simulink model "Simulink_mg_1234_with_DistributedControl_ControlConmutado"  (R2018a)
settings: Solver=VariableStepAuto  StartTime=0.0  StopTime=50  FixedStep=1e-6  MaxStep=1e-3  RelTol=1e-3
values from neighbouring files (symbols this model uses):
  aij = 1    [Simulation_Base_4_mg.m]    (also in Simulation_alpha_vs_tau.m)
  aij_1 = 10    [Simulation_Base_4_mg.m]    (also in Simulation_alpha_vs_tau.m)
  aij_2 = 10    [Simulation_Base_4_mg.m]    (also in Simulation_alpha_vs_tau.m)
  aij_3 = 10    [Simulation_Base_4_mg.m]    (also in Simulation_alpha_vs_tau.m)
  aij_4 = 10    [Simulation_Base_4_mg.m]    (also in Simulation_alpha_vs_tau.m)
  C_mg_1 = Ctot .* dist    [Simulation_Base_4_mg.m]    (also in Simulation_alpha_vs_tau.m)
  C_mg_2 = Ctot .* dist    [Simulation_Base_4_mg.m]    (also in Simulation_alpha_vs_tau.m)
  C_mg_3 = Ctot .* dist    [Simulation_Base_4_mg.m]    (also in Simulation_alpha_vs_tau.m)
  C_mg_4 = Ctot .* dist    [Simulation_Base_4_mg.m]    (also in Simulation_alpha_vs_tau.m)
  g12 = 1.2    [Simulation_Base_4_mg.m]    (also in Simulation_alpha_vs_tau.m)
  g12_1 = 1/r_jk    (= 10)    [Simulation_Base_4_mg.m]    (also in Simulation_alpha_vs_tau.m)
  g12_2 = 1/r_jk    (= 10)    [Simulation_Base_4_mg.m]    (also in Simulation_alpha_vs_tau.m)
  g12_3 = 1/r_jk    (= 10)    [Simulation_Base_4_mg.m]    (also in Simulation_alpha_vs_tau.m)
  g12_4 = 1/r_jk    (= 10)    [Simulation_Base_4_mg.m]    (also in Simulation_alpha_vs_tau.m)
  g13 = ((0.383+1.756) / (0.383*1.756))^(-1)    (= 0.31442169238)    [Simulation_Base_4_mg.m]    (also in Simulation_alpha_vs_tau.m)
  g13_1 = 1/r_jk    (= 10)    [Simulation_Base_4_mg.m]    (also in Simulation_alpha_vs_tau.m)
  g13_3 = 1/r_jk    (= 10)    [Simulation_Base_4_mg.m]    (also in Simulation_alpha_vs_tau.m)
  g13_4 = 1/r_jk    (= 10)    [Simulation_Base_4_mg.m]    (also in Simulation_alpha_vs_tau.m)
  g23_1 = 1/r_jk    (= 10)    [Simulation_Base_4_mg.m]    (also in Simulation_alpha_vs_tau.m)
  g23_4 = 1/r_jk    (= 10)    [Simulation_Base_4_mg.m]    (also in Simulation_alpha_vs_tau.m)
  g24 = 1.55    [Simulation_Base_4_mg.m]    (also in Simulation_alpha_vs_tau.m)
  g24_3 = 1/r_jk    (= 10)    [Simulation_Base_4_mg.m]    (also in Simulation_alpha_vs_tau.m)
  g24_4 = 1/r_jk    (= 10)    [Simulation_Base_4_mg.m]    (also in Simulation_alpha_vs_tau.m)
  g34 = 0.75    [Simulation_Base_4_mg.m]    (also in Simulation_alpha_vs_tau.m)
  g34_3 = 1/r_jk    (= 10)    [Simulation_Base_4_mg.m]    (also in Simulation_alpha_vs_tau.m)
  g34_4 = 1/r_jk    (= 10)    [Simulation_Base_4_mg.m]    (also in Simulation_alpha_vs_tau.m)
  h = 0.99    [Simulation_Base_4_mg.m]    (also in Simulation_alpha_vs_tau.m)
  I_rate = [100,50,33,33]    [Simulation_Base_4_mg.m]    (also in Simulation_alpha_vs_tau.m)
  I_rate_1 = [5, 2.5, 2.5]    [Simulation_Base_4_mg.m]    (also in Simulation_alpha_vs_tau.m)
  I_rate_2 = [2.5, 5]    [Simulation_Base_4_mg.m]    (also in Simulation_alpha_vs_tau.m)
  I_rate_3 = [4, 3, 2, 1]    [Simulation_Base_4_mg.m]    (also in Simulation_alpha_vs_tau.m)
  I_rate_4 = [4, 3, 2, 1]    [Simulation_Base_4_mg.m]    (also in Simulation_alpha_vs_tau.m)
  k_ii = 60    [Simulation_Base_4_mg.m]    (also in Simulation_alpha_vs_tau.m)
  k_ii2 = 10    [Simulation_Base_4_mg.m]    (also in Simulation_alpha_vs_tau.m)
  k_ii_1 = 1000    [Simulation_Base_4_mg.m]    (also in Simulation_alpha_vs_tau.m)
  k_ii_2 = 1000    [Simulation_Base_4_mg.m]    (also in Simulation_alpha_vs_tau.m)
  k_ii_3 = 1000    [Simulation_Base_4_mg.m]    (also in Simulation_alpha_vs_tau.m)
  k_ii_4 = 1000    [Simulation_Base_4_mg.m]    (also in Simulation_alpha_vs_tau.m)
  k_iv = 3    [Simulation_Base_4_mg.m]    (also in Simulation_alpha_vs_tau.m = 1)
  k_iv_1 = 30    [Simulation_Base_4_mg.m]    (also in Simulation_alpha_vs_tau.m)
  k_iv_2 = 30    [Simulation_Base_4_mg.m]    (also in Simulation_alpha_vs_tau.m)
  k_iv_3 = 30    [Simulation_Base_4_mg.m]    (also in Simulation_alpha_vs_tau.m)
  k_iv_4 = 30    [Simulation_Base_4_mg.m]    (also in Simulation_alpha_vs_tau.m)
  k_pi = 30    [Simulation_Base_4_mg.m]    (also in Simulation_alpha_vs_tau.m = 25)
  k_pi2 = 0.5    [Simulation_Base_4_mg.m]    (also in Simulation_alpha_vs_tau.m)
  k_pi_1 = 10    [Simulation_Base_4_mg.m]    (also in Simulation_alpha_vs_tau.m)
  k_pi_2 = 10    [Simulation_Base_4_mg.m]    (also in Simulation_alpha_vs_tau.m)
  k_pi_3 = 10    [Simulation_Base_4_mg.m]    (also in Simulation_alpha_vs_tau.m)
  k_pi_4 = 10    [Simulation_Base_4_mg.m]    (also in Simulation_alpha_vs_tau.m)
  kd_1 = [5, 2.5, 2.5]    [Simulation_Base_4_mg.m]    (also in Simulation_alpha_vs_tau.m)
  kd_2 = [2.5, 50]    [Simulation_Base_4_mg.m]    (also in Simulation_alpha_vs_tau.m)
  kd_3 = [4, 3, 2, 1]    [Simulation_Base_4_mg.m]    (also in Simulation_alpha_vs_tau.m)
  kd_4 = [4, 3, 2, 1]    [Simulation_Base_4_mg.m]    (also in Simulation_alpha_vs_tau.m)
  L_mg_1 = ones(n) .* n .* Ltot    [Simulation_Base_4_mg.m]    (also in Simulation_alpha_vs_tau.m)
  L_mg_2 = ones(n) .* n .* Ltot    [Simulation_Base_4_mg.m]    (also in Simulation_alpha_vs_tau.m)
  L_mg_3 = ones(n) .* n .* Ltot    [Simulation_Base_4_mg.m]    (also in Simulation_alpha_vs_tau.m)
  L_mg_4 = ones(n) .* n .* Ltot    [Simulation_Base_4_mg.m]    (also in Simulation_alpha_vs_tau.m)
  P_load_vertex_1 = [   P_load_vertex_1;                                                 P_aux(i1,1) , P_aux(i2,2) , P_aux(i3,3) ]    [Simulation_Base_4_mg.m]    (also in Simulation_alpha_vs_tau.m)
  P_load_vertex_2 = [   P_load_vertex_2;                                                 P_aux(i1,1) , P_aux(i2,2) ]    [Simulation_Base_4_mg.m]    (also in Simulation_alpha_vs_tau.m)
  P_load_vertex_3 = [   P_load_vertex_3;                                                 P_aux(i1,1) , P_aux(i2,2) , P_aux(i3,3), P_aux(i4,4) ]    [Simulation_Base_4_mg.m]    (also in Simulation_alpha_vs_tau.m)
  P_load_vertex_4 = [   P_load_vertex_4;                                                 P_aux(i1,1) , P_aux(i2,2) , P_aux(i3,3), P_aux(i4,4) ]    [Simulation_Base_4_mg.m]    (also in Simulation_alpha_vs_tau.m)
  r_d0 = 1.3    [Simulation_Base_4_mg.m]    (also in Simulation_alpha_vs_tau.m)
  rd_mg_1 = n^2 * rtot .* dist    [Simulation_Base_4_mg.m]    (also in Simulation_alpha_vs_tau.m)
  rd_mg_2 = n^2 * rtot .* dist    [Simulation_Base_4_mg.m]    (also in Simulation_alpha_vs_tau.m)
  rd_mg_3 = n^2 * rtot .* dist    [Simulation_Base_4_mg.m]    (also in Simulation_alpha_vs_tau.m)
  rd_mg_4 = n^2 * rtot .* dist    [Simulation_Base_4_mg.m]    (also in Simulation_alpha_vs_tau.m)
  tau = 0.5    [Simulation_Base_4_mg.m]    (also in Simulation_alpha_vs_tau.m = 0.066)
  time_1 = 0.5    [Simulation_Base_4_mg.m]    (also in Simulation_alpha_vs_tau.m)
  time_2 = 15    [Simulation_Base_4_mg.m]    (also in Simulation_alpha_vs_tau.m = 5)
  time_4 = 5    [Simulation_Base_4_mg.m]    (also in Simulation_alpha_vs_tau.m = 15)
  time_6 = 50    [Simulation_Base_4_mg.m]    (also in Simulation_alpha_vs_tau.m = 13)
  time_7 = 50    [Simulation_Base_4_mg.m]    (also in Simulation_alpha_vs_tau.m = 100)
  time_8 = 50    [Simulation_Base_4_mg.m]    (also in Simulation_alpha_vs_tau.m = 100)
  time_9 = 100    [Simulation_Base_4_mg.m]    (also in Simulation_alpha_vs_tau.m)
  time_a_down = 100    [Simulation_alpha_vs_tau.m]
  time_a_up = 100    [Simulation_alpha_vs_tau.m]
  time_tau_down = 25    [Simulation_alpha_vs_tau.m]
  V_ref = 1050    [Simulation_Base_4_mg.m]    (also in Simulation_alpha_vs_tau.m)
undefined symbols (not defined in the file or in its folder): Zout_den_source, Zout_num_source
libraries: fl_lib x128, nesl_utility x89, elec_lib x26
(part 2 of 2)

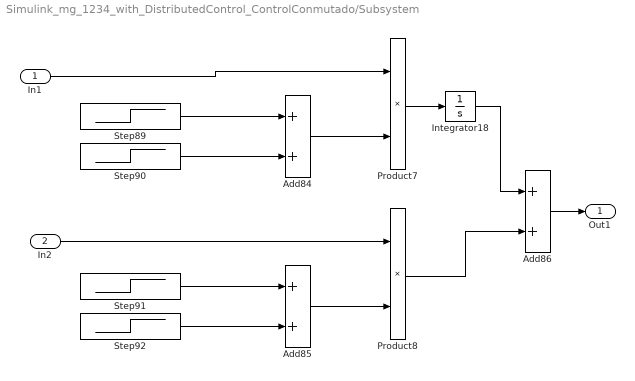
== system Simulink_mg_1234_with_DistributedControl_ControlConmutado/Subsystem ==
  In1 : Inport
  In2 : Inport  Port=2
  Add84 : Sum
  Add85 : Sum
  Add86 : Sum
  Integrator18 : Integrator
  Product7 : Product
  Product8 : Product
  Step89 : Step  Time=time_8  Before=k_ii  After=k_ii2  SampleTime=0
  Step90 : Step  Time=time_9  SampleTime=0
  Step91 : Step  Time=time_8  Before=k_pi  After=k_pi2  SampleTime=0
  Step92 : Step  Time=time_9  SampleTime=0
  Out1 : Outport
  wires:
  Integrator18/1 -> Add86/1
  Step92/1 -> Add85/2
  Add85/1 -> Product8/2
  Step89/1 -> Add84/1
  Step90/1 -> Add84/2
  Step91/1 -> Add85/1
  Add84/1 -> Product7/2
  Product7/1 -> Integrator18/1
  Product8/1 -> Add86/2
  In2/1 -> Product8/1
  In1/1 -> Product7/1
  Add86/1 -> Out1/1

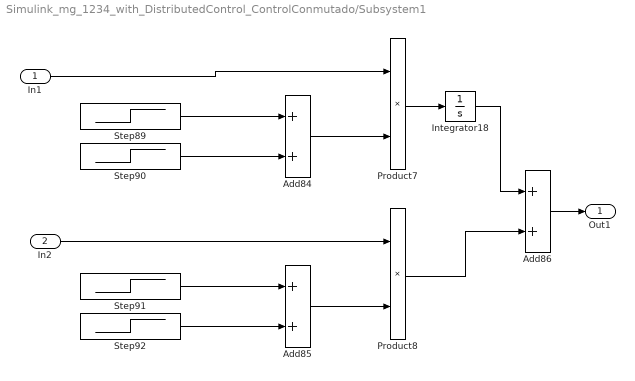
== system Simulink_mg_1234_with_DistributedControl_ControlConmutado/Subsystem1 ==
  In1 : Inport
  In2 : Inport  Port=2
  Add84 : Sum
  Add85 : Sum
  Add86 : Sum
  Integrator18 : Integrator
  Product7 : Product
  Product8 : Product
  Step89 : Step  Time=time_8  Before=k_ii  After=k_ii2  SampleTime=0
  Step90 : Step  Time=time_9  SampleTime=0
  Step91 : Step  Time=time_8  Before=k_pi  After=k_pi2  SampleTime=0
  Step92 : Step  Time=time_9  SampleTime=0
  Out1 : Outport
  wires:
  Add86/1 -> Out1/1
  In1/1 -> Product7/1
  In2/1 -> Product8/1
  Product8/1 -> Add86/2
  Product7/1 -> Integrator18/1
  Add84/1 -> Product7/2
  Step91/1 -> Add85/1
  Step90/1 -> Add84/2
  Step89/1 -> Add84/1
  Add85/1 -> Product8/2
  Step92/1 -> Add85/2
  Integrator18/1 -> Add86/1

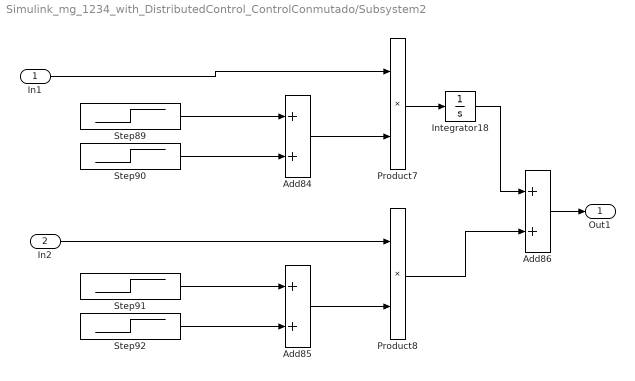
== system Simulink_mg_1234_with_DistributedControl_ControlConmutado/Subsystem2 ==
  In1 : Inport
  In2 : Inport  Port=2
  Add84 : Sum
  Add85 : Sum
  Add86 : Sum
  Integrator18 : Integrator
  Product7 : Product
  Product8 : Product
  Step89 : Step  Time=time_8  Before=k_ii  After=k_ii2  SampleTime=0
  Step90 : Step  Time=time_9  SampleTime=0
  Step91 : Step  Time=time_8  Before=k_pi  After=k_pi2  SampleTime=0
  Step92 : Step  Time=time_9  SampleTime=0
  Out1 : Outport
  wires:
  Add86/1 -> Out1/1
  In1/1 -> Product7/1
  In2/1 -> Product8/1
  Product8/1 -> Add86/2
  Product7/1 -> Integrator18/1
  Add84/1 -> Product7/2
  Step91/1 -> Add85/1
  Step90/1 -> Add84/2
  Step89/1 -> Add84/1
  Add85/1 -> Product8/2
  Step92/1 -> Add85/2
  Integrator18/1 -> Add86/1

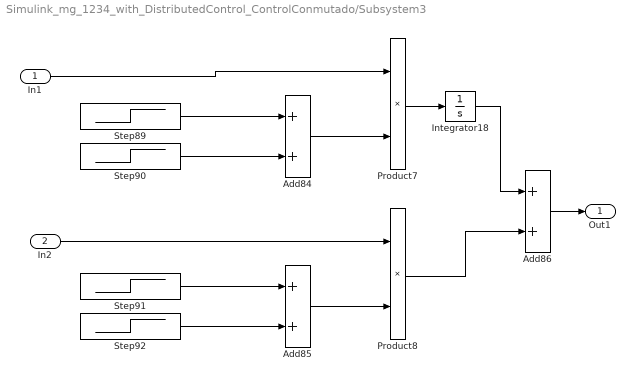
== system Simulink_mg_1234_with_DistributedControl_ControlConmutado/Subsystem3 ==
  In1 : Inport
  In2 : Inport  Port=2
  Add84 : Sum
  Add85 : Sum
  Add86 : Sum
  Integrator18 : Integrator
  Product7 : Product
  Product8 : Product
  Step89 : Step  Time=time_8  Before=k_ii  After=k_ii2  SampleTime=0
  Step90 : Step  Time=time_9  SampleTime=0
  Step91 : Step  Time=time_8  Before=k_pi  After=k_pi2  SampleTime=0
  Step92 : Step  Time=time_9  SampleTime=0
  Out1 : Outport
  wires:
  Integrator18/1 -> Add86/1
  Step92/1 -> Add85/2
  Add85/1 -> Product8/2
  Step89/1 -> Add84/1
  Step90/1 -> Add84/2
  Step91/1 -> Add85/1
  Add84/1 -> Product7/2
  Product7/1 -> Integrator18/1
  Product8/1 -> Add86/2
  In2/1 -> Product8/1
  In1/1 -> Product7/1
  Add86/1 -> Out1/1

== matlab function Simulink_mg_1234_with_DistributedControl_ControlConmutado/MATLAB Function1 ==
  data: i input; error_1 output; error_2 output; error_3 output; error_4 output; aij input
function [error_1,error_2,error_3, error_4] = fcn(i, aij)


%aij = 30;
%Connection matrix
AG = [  0 aij aij aij ; ...
        aij 0 aij aij ; ...
        aij aij 0 aij ;...
        aij aij aij 0]; %Communication matrices
n = 4;
i_int = i';
AG1 = AG - eye(n);
%sum_a = sum(AG1');
sum_a = sum(AG');
%AG1 = AG1 * i_int';
AG = AG * i_int';


%error = sum_a .* i_int - AG1';
error = sum_a .* i_int - AG';
error_1 = -error(1); 
error_2 = -error(2);
error_3 = -error(3); 
error_4 = -error(4);

== matlab function Simulink_mg_1234_with_DistributedControl_ControlConmutado/MATLAB Function2 ==
  data: i input; error_1 output; error_2 output; error_3 output; error_4 output; aij input
function [error_1,error_2,error_3, error_4] = fcn(i, aij)


%aij = 30;
%Connection matrix
AG = [  0 aij aij  aij ; ...
        aij 0 aij aij ; ...
        aij aij 0 aij ;...
        aij aij aij 0]; %Communication matrices
n = 4;
i_int = i';
AG1 = AG - eye(n);
%sum_a = sum(AG1');
sum_a = sum(AG');
%AG1 = AG1 * i_int';
AG = AG * i_int';


%error = sum_a .* i_int - AG1';
error = sum_a .* i_int - AG';
error_1 = -error(1); 
error_2 = -error(2);
error_3 = -error(3); 
error_4 = -error(4);

== matlab function Simulink_mg_1234_with_DistributedControl_ControlConmutado/MATLAB Function3 ==
  data: i input; error_1 output; error_2 output; error_3 output; aij input
function [error_1,error_2,error_3] = fcn(i, aij)


%aij = 30;
%Connection matrix
AG = [  0 aij aij ; ...
        aij 0 aij; ...
        aij aij 0  ]; %Communication matrices
n = 3;
i_int = i';
AG1 = AG - eye(n);
%sum_a = sum(AG1');
sum_a = sum(AG');
%AG1 = AG1 * i_int';
AG = AG * i_int';


%error = sum_a .* i_int - AG1';
error = sum_a .* i_int - AG';
error_1 = -error(1); 
error_2 = -error(2);
error_3 = -error(3);

== matlab function Simulink_mg_1234_with_DistributedControl_ControlConmutado/MATLAB Function4 ==
  data: i input; error_1 output; error_2 output; aij input
function [error_1,error_2] = fcn(i, aij)


%aij = 30;
%Connection matrix
AG = [  0 aij ; ...
        aij 0 ]; %Communication matrices
n = 2;
i_int = i';
AG1 = AG - eye(n);
%sum_a = sum(AG1');
sum_a = sum(AG');
%AG1 = AG1 * i_int';
AG = AG * i_int';


%error = sum_a .* i_int - AG1';
error = sum_a .* i_int - AG';
error_1 = -error(1); 
error_2 = -error(2);

== matlab function Simulink_mg_1234_with_DistributedControl_ControlConmutado/MATLAB Function5 ==
  data: i input; error_1 output; error_2 output; error_3 output; aij input; error_4 output
function [error_1,error_2,error_3, error_4] = fcn(i, aij)


%aij = 30;
%Connection matrix
AG = [  0 aij 0  0; ...
        aij 0 aij 0; ...
        0 aij 0  aij;...
        0 0   aij 0 ]; %Communication matrices
n = 4;
i_int = i';
AG1 = AG - eye(n);
%sum_a = sum(AG1');
sum_a = sum(AG');
%AG1 = AG1 * i_int';
AG = AG * i_int';


%error = sum_a .* i_int - AG1';
error = sum_a .* i_int - AG';
error_1 = -error(1); 
error_2 = -error(2);
error_3 = -error(3); 
error_4 = -error(4);
